simulink model "general_model"  (R2024b)
settings: Solver=VariableStepAuto  StartTime=0.0  StopTime=Tsim  RelTol=1e-3
values from neighbouring files (symbols this model uses):
  ap_t = 0    [P1.m]
  as_t = as    [P1.m]
  Da0_t = 0    [P1.m]
  Ga = 0.095    [P1.m]
  Gf = 1    [P1.m]
  Gs = 1    [P1.m]
  R0_t = 0    [P1.m]
  wp_plus = 0.02    [P1.m]
  ws_minus = 40    [P1.m]
libraries: cstblocks x2, simulink x1
settings Model: Creator=lucap  LastModifiedBy=lucap

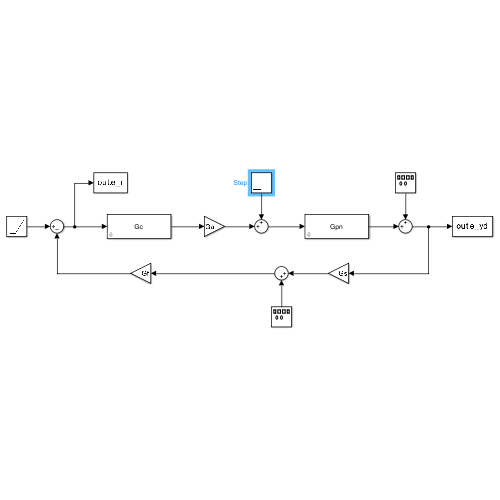
[thumbnail: Simulink's stored preview of the top-level diagram]
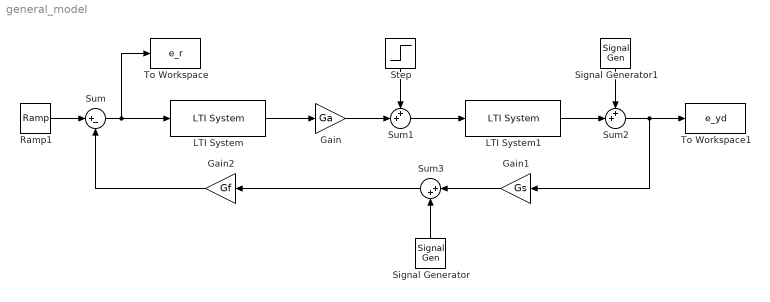
== system general_model ==
  Gain : Gain  Gain=Ga
  Gain1 : Gain  Gain=Gs
  Gain2 : Gain  Gain=Gf
  LTI System : cstblocks/LTI System  sys=Gc  IC=[]  PadeOrder=0
  LTI System1 : cstblocks/LTI System  sys=Gpn  IC=[]  PadeOrder=0
  Ramp1 : simulink/Sources/Ramp  slope=R0_t  start=0  InitialOutput=0
  Signal Generator : SignalGenerator  Amplitude=as_t  Frequency=ws_minus  Units=rad/sec
  Signal Generator1 : SignalGenerator  Amplitude=ap_t  Frequency=wp_plus  Units=rad/sec
  Step : Step  Time=0  After=Da0_t  SampleTime=0
  Sum : Sum  Inputs=|+-
  Sum1 : Sum  Inputs=++|
  Sum2 : Sum  Inputs=++|
  Sum3 : Sum  Inputs=|++
  To Workspace : ToWorkspace  VariableName=e_r  SaveFormat=Timeseries  SampleTime=-1
  To Workspace1 : ToWorkspace  VariableName=e_yd  SaveFormat=Timeseries  SampleTime=-1
  wires:
  Sum2/1 -> Gain1/1, To Workspace1/1
  Signal Generator1/1 -> Sum2/1
  Gain1/1 -> Sum3/1
  LTI System1/1 -> Sum2/2
  Sum1/1 -> LTI System1/1
  Gain2/1 -> Sum/2
  Step/1 -> Sum1/1
  Sum/1 -> To Workspace/1, LTI System/1
  Ramp1/1 -> Sum/1
  Signal Generator/1 -> Sum3/2
  LTI System/1 -> Gain/1
  Sum3/1 -> Gain2/1
  Gain/1 -> Sum1/2
